simulink model "dof3_new_2023a"  (R2022b)
settings: Solver=ode5  StartTime=0.0  StopTime=100  FixedStep=0.001  RelTol=1e-3
InitFcn:
  | % 整车参数
  | % 定义车辆参数
  | m = 1370 + 89.9 + 65.2 + 22*4;       % 车辆质量 (kg)
  | % Vx = 120/3.6;        % 纵向速度 (m/s)
  | Cf = -4.487763550086564e+04 * 2;    % 前轴总侧偏刚度 (N/rad)
  | Cr = Cf;   % 后轴总侧偏刚度 (N/rad)
  | lf = 1.11;       % 质心到前轴距离 (m)
  | lr = 2.866-lf;       % 质心到后轴距离 (m)
  | Iz = 2315.3 + 0.08 + 0.08 + 0.8*4;      % 绕z轴转动惯量 (kg·m²)
  | Bf = 1.55;
  | Br = 1.55;
  | Re = 0.325;
libraries: simulink_extras x4, Solver_SF x1, simulink x1
settings Model: Creator=23649  LastModifiedBy=23649
settings OptimizationCC: ReuseModelBlockBuffer=on
settings RTWCC: GPUComputeCapability=5.0
settings ConfigComp: CovBoundaryAbsTol=1.0e-5

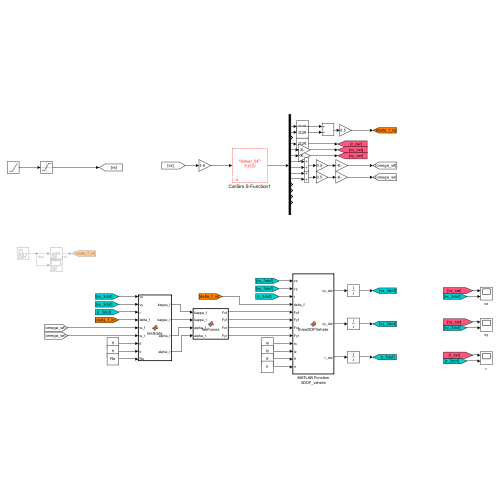
[thumbnail: Simulink's stored preview of the top-level diagram]
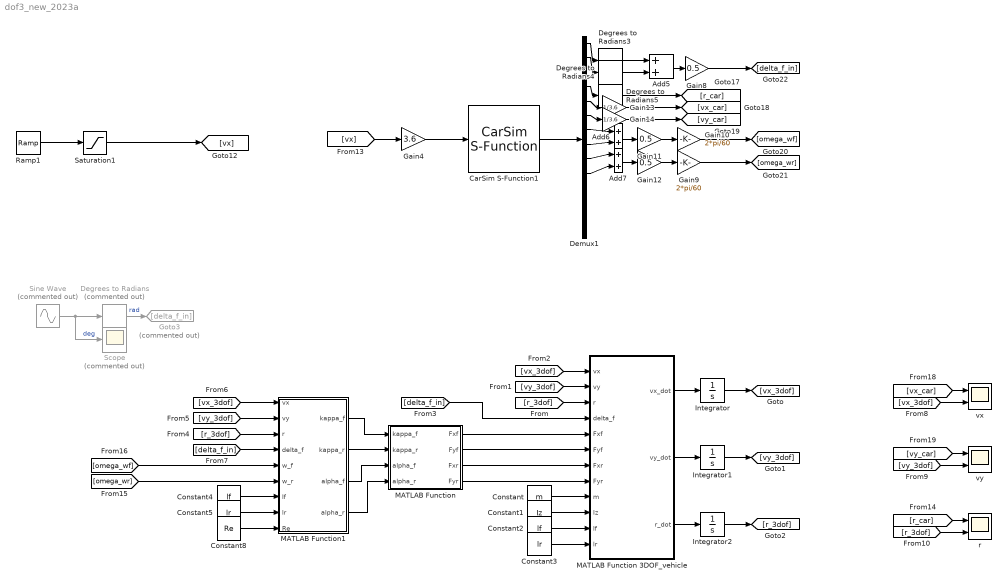
== system dof3_new_2023a ==
  Add5 : Sum
  Add6 : Sum
  Add7 : Sum
  CarSim S-Function1 : Solver_SF/CarSim S-Function  Priority=1  SIMFILE=simfile.sim  Run_RTs=off  vs_state_ind=Run  StopMode_ind=Vehicle Model
  Constant : Constant  Value=m
  Constant1 : Constant  Value=Iz
  Constant2 : Constant  Value=lf
  Constant3 : Constant  Value=lr
  Constant4 : Constant  Value=lf
  Constant5 : Constant  Value=lr
  Constant8 : Constant  Value=Re
  Degrees to Radians : simulink_extras/Transformations/Degrees to Radians  Commented=on
  Degrees to Radians3 : simulink_extras/Transformations/Degrees to Radians
  Degrees to Radians4 : simulink_extras/Transformations/Degrees to Radians
  Degrees to Radians5 : simulink_extras/Transformations/Degrees to Radians
  Demux1 : Demux  Outputs=14
  Gain10 : Gain  Gain=2*pi/60
  Gain11 : Gain  Gain=0.5
  Gain12 : Gain  Gain=0.5
  Gain13 : Gain  Gain=1/3.6
  Gain14 : Gain  Gain=1/3.6
  Gain4 : Gain  Gain=3.6
  Gain8 : Gain  Gain=0.5
  Gain9 : Gain  Gain=2*pi/60
  Goto3 : Goto  Commented=on  GotoTag=delta_f_in
  Integrator : Integrator
  Integrator1 : Integrator
  Integrator2 : Integrator
  MATLAB Function : MATLAB Function  TreatAsAtomicUnit=on
  MATLAB Function 3DOF_vehicle : MATLAB Function  TreatAsAtomicUnit=on
  MATLAB Function1 : MATLAB Function  TreatAsAtomicUnit=on
  Ramp1 : simulink/Sources/Ramp  slope=5  start=0  InitialOutput=0
  Saturation1 : Saturate  UpperLimit=15
  Scope : Scope  Commented=on
  Sine Wave : Sin  Commented=on  Amplitude=5  SampleTime=0
  r : Scope  NumInputPorts=2
  vx : Scope  NumInputPorts=2
  vy : Scope  NumInputPorts=2
  wires:
  MATLAB Function 3DOF_vehicle/1(vx_dot) -> Integrator/1
  MATLAB Function 3DOF_vehicle/3(r_dot) -> Integrator2/1
  MATLAB Function 3DOF_vehicle/2(vy_dot) -> Integrator1/1
  Integrator/1 -> [vx_3dof]
  Integrator1/1 -> [vy_3dof]
  Integrator2/1 -> [r_3dof]
  [vx_3dof] -> MATLAB Function 3DOF_vehicle/1(vx)
  [r_3dof] -> MATLAB Function 3DOF_vehicle/3(r)
  [vy_3dof] -> MATLAB Function 3DOF_vehicle/2(vy)
  [delta_f_in] -> MATLAB Function 3DOF_vehicle/4(delta_f)
  MATLAB Function/1(Fxf) -> MATLAB Function 3DOF_vehicle/5(Fxf)
  MATLAB Function/2(Fyf) -> MATLAB Function 3DOF_vehicle/6(Fyf)
  MATLAB Function/3(Fxr) -> MATLAB Function 3DOF_vehicle/7(Fxr)
  MATLAB Function/4(Fyr) -> MATLAB Function 3DOF_vehicle/8(Fyr)
  Constant/1 -> MATLAB Function 3DOF_vehicle/9(m)
  Constant3/1 -> MATLAB Function 3DOF_vehicle/12(lr)
  Constant2/1 -> MATLAB Function 3DOF_vehicle/11(lf)
  Constant1/1 -> MATLAB Function 3DOF_vehicle/10(Iz)
  MATLAB Function1/1(kappa_f) -> MATLAB Function/1(kappa_f)
  MATLAB Function1/4(alpha_r) -> MATLAB Function/4(alpha_r)
  MATLAB Function1/2(kappa_r) -> MATLAB Function/2(kappa_r)
  MATLAB Function1/3(alpha_f) -> MATLAB Function/3(alpha_f)
  [vx_3dof] -> MATLAB Function1/1(vx)
  [vy_3dof] -> MATLAB Function1/2(vy)
  [r_3dof] -> MATLAB Function1/3(r)
  [delta_f_in] -> MATLAB Function1/4(delta_f)
  [omega_wf] -> MATLAB Function1/5(w_f)
  [omega_wr] -> MATLAB Function1/6(w_r)
  Constant4/1 -> MATLAB Function1/7(lf)
  Constant5/1 -> MATLAB Function1/8(lr)
  Sine Wave/1 -> Degrees to Radians/1, Scope/1  "deg"
  Degrees to Radians/1 -> Goto3/1  "rad"
  [vx_3dof] -> vx/2
  [vy_3dof] -> vy/2
  [r_3dof] -> r/2
  Constant8/1 -> MATLAB Function1/9(Re)
  [r_car] -> r/1
  [vy_car] -> vy/1
  [vx_car] -> vx/1
  [vx] -> Gain4/1
  CarSim S-Function1/1 -> Demux1/1
  Ramp1/1 -> Saturation1/1
  Saturation1/1 -> [vx]
  Gain4/1 -> CarSim S-Function1/1
  Demux1/1 -> Degrees to Radians3/1
  Demux1/2 -> Degrees to Radians4/1
  Add5/1 -> Gain8/1
  Gain8/1 -> [delta_f_in]
  Demux1/4 -> Degrees to Radians5/1
  Demux1/5 -> Gain13/1
  Demux1/6 -> Gain14/1
  Gain9/1 -> [omega_wr]
  Gain12/1 -> Gain9/1
  Add7/1 -> Gain12/1
  Add6/1 -> Gain11/1
  Gain11/1 -> Gain10/1
  Gain10/1 -> [omega_wf]
  Demux1/8 -> Add6/2
  Demux1/7 -> Add6/1
  Demux1/9 -> Add7/1
  Demux1/10 -> Add7/2
  Degrees to Radians3/1 -> Add5/1
  Degrees to Radians4/1 -> Add5/2
  Degrees to Radians5/1 -> [r_car]
  Gain13/1 -> [vx_car]
  Gain14/1 -> [vy_car]

== matlab function dof3_new_2023a/MATLAB Function ==
  data: kappa_f input; Fxf output; Fyf output; Fxr output; Fyr output; kappa_r input; alpha_f input; alpha_r input
function [Fxf, Fyf, Fxr, Fyr] = tireForces(kappa_f, kappa_r, alpha_f, alpha_r)
    %% 轮胎力
    % 轮胎刚度
    Cxf =  37500*2;
    Cyf = -90000 * 2;
    
    Cxr = Cxf;
    Cyr = Cyf;
    
    % 前轴纵侧向
    Fxf = Cxf * kappa_f;
    Fyf = Cyf * alpha_f;

    % 后轴纵侧向
    Fxr = Cxr * kappa_r;
    Fyr = Cyr * alpha_r;

    % 物理极限
    [Fxf, Fyf] = limitedTireForce(Fxf, Fyf);
    [Fxr, Fyr] = limitedTireForce(Fxr, Fyr);

end

function [Fx, Fy] = limitedTireForce(Fx, Fy)

    Fmax =  (1370 + 89.9 + 65.2 + 22*4) * 9.8/2;

    if (Fx^2 + Fy^2) > Fmax^2
        wx = Fx/sqrt(Fx^2 + Fy^2);
        wy = Fy/sqrt(Fx^2 + Fy^2);
        Fx = wx*Fmax;
        Fy = wy*Fmax;
    end

end

== matlab function dof3_new_2023a/MATLAB Function 3DOF_vehicle ==
  data: vx input; vy input; r input; delta_f input; Fxf input; Fyf input; Fxr input; Fyr input; vx_dot output; vy_dot output; r_dot output; m input; Iz input; lf input; lr input
function [vx_dot, vy_dot, r_dot] =  threeDOFVehicle(vx, vy, r, delta_f, Fxf, Fyf, Fxr, Fyr, m, Iz, lf, lr)
    % 纵向风阻力
    A = 2.2;
    D = 1.206;
    CFx = 0.3;
    Fxair = 1/2 * CFx * D * A * vx*abs(vx);
    
    %% 3dof 整车平面运动动力学模型
    % 纵向
    vx_dot = vy*r + (Fxf*cos(delta_f) - Fyf*sin(delta_f) + Fxr - Fxair) / m;
    
    % 侧向
    vy_dot = -vx*r + (Fxf*sin(delta_f) + Fyf*cos(delta_f) + Fyr) / m;

    % 横摆
    r_dot = (lf*(Fxf*sin(delta_f) + Fyf*cos(delta_f)) - lr*Fyr) / Iz;
end

== matlab function dof3_new_2023a/MATLAB Function1 ==
  data: vx input; vy input; r input; delta_f input; w_f input; w_r input; lf input; kappa_f output; kappa_r output; lr input; alpha_f output; alpha_r output; Re input
function [kappa_f, kappa_r, alpha_f, alpha_r] = tireState(vx, vy, r, delta_f, w_f, w_r, lf, lr, Re)
    % 轮胎状态
    % - alpha
    % - kappa
    Bf = 0;
    Br = 0;

    delta_r = 0;

    [kappa_f, alpha_f] = ka_figure(vx, vy, r, delta_f, w_f, Bf, lf, Re);
    [kappa_r, alpha_r] = ka_figure(vx, vy, r, delta_r, w_r, Br, -lr, Re);


end

function [kappa, alpha] = ka_figure(vx, vy, r, delta, w, B, l, Re)
    vwx_V = vx - B/2 * r;
    vwy_V = vy + l * r;

    vwx_W = vwx_V*cos(delta) + vwy_V*sin(delta);
    vwy_W = -vwx_V*sin(delta) + vwy_V*cos(delta);

    vwx_W_nozero = vwx_W;
    if abs(vwx_W_nozero) < 1e-5
        vwx_W_nozero = 1e-5;
    end

    alpha = atan(vwy_W / vwx_W_nozero);
    kappa = (Re*w - vwx_W) / abs(vwx_W_nozero);
end
